simulink model "Ex6_6"  (Simulink 6.0)
settings: Solver=FixedStepDiscrete  SolverMode=SingleTasking  StartTime=0.0  StopTime=Ts*10  FixedStep=Ts  RelTol=1e-3  AbsTol=1e-6
values from neighbouring files (symbols this model uses):
  alpha1 = 1-1/Gain1    (= 0.99999)    [Ex6_6Launch.m]
  alpha2 = 1-1/Gain2    (= 0.99999)    [Ex6_6Launch.m]
  Ampl = 10^(Amp_dB/20)-pi/1024    (= 0.498119272052)    [Ex6_6Launch.m]
  finrad = Fin*2*pi    (= 882038.953034)    [Ex6_6Launch.m]
  GBW1 = 30000e6    (= 30000000000)    [Ex6_6Launch.m]
  GBW2 = 100e6    (= 100000000)    [Ex6_6Launch.m]
  sr1 = 79e6    (= 79000000)    [Ex6_6Launch.m]
  sr2 = 325e6    (= 325000000)    [Ex6_6Launch.m]
  Ts = 1/Fs    (= 2e-08)    [Ex6_6Launch.m]
undefined symbols (not defined in the file or in its folder): slew
settings Model: Creator=francomaloberti  LastModifiedBy=Cri  ExtModeAutoUpdateStatusClock=off
settings DataIOCC: LimitDataPoints=off  SignalLoggingName=sigsOut
settings OptimizationCC: BooleanDataType=off  InlineInvariantSignals=off
settings DebuggingCC: SolverPrmCheckMsg=none
settings HardwareCC: TargetUnknown=on

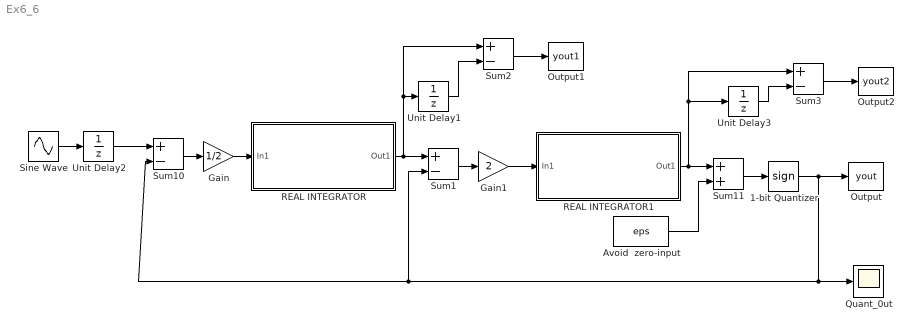
== system Ex6_6 ==
  1-bit Quantizer : Signum
  Avoid  zero-input : Constant  Value=eps
  Gain : Gain  Gain=1/2  SaturateOnIntegerOverflow=on
  Gain1 : Gain  Gain=2  SaturateOnIntegerOverflow=on
  Output : ToWorkspace  VariableName=yout  SampleTime=-1  SaveFormat=Array
  Output1 : ToWorkspace  VariableName=yout1  SampleTime=-1  SaveFormat=Array
  Output2 : ToWorkspace  VariableName=yout2  SampleTime=-1  SaveFormat=Array
  Quant_0ut : Scope
  REAL INTEGRATOR : Subsystem
      mask Display:
      | patch([10 40 10 10], [0 20 40 0],[1 0 1])
      | plot([10 40 10 10], [0 20 40 0])
      | plot([0 10], [20 20])
      | dpoly([0 1], [1 -1], 'z-')
      | port_label('input', 1, 'in')
  REAL INTEGRATOR1 : Subsystem
      mask Display:
      | patch([10 40 10 10], [0 20 40 0],[1 0 1])
      | plot([10 40 10 10], [0 20 40 0])
      | plot([0 10], [20 20])
      | dpoly([0 1], [1 -1], 'z-')
      | port_label('input', 1, 'in')
  Sine Wave : Sin  Amplitude=Ampl  Frequency=finrad  SampleTime=0
  Sum{1..3,10} (4 alike) : Sum  Inputs=+-  SaturateOnIntegerOverflow=on  InputSameDT=on
  Sum11 : Sum  SaturateOnIntegerOverflow=on  InputSameDT=on
  Unit Delay1 : UnitDelay  SampleTime=Ts
  Unit Delay2 : UnitDelay  SampleTime=Ts
  Unit Delay3 : UnitDelay  SampleTime=Ts
  wires:
  Sine Wave/1 -> Unit Delay2/1
  Unit Delay2/1 -> Sum10/1
  1-bit Quantizer/1 -> Quant_0ut/1, Sum10/2, Sum1/2, Output/1
  Sum10/1 -> Gain/1
  Gain/1 -> REAL INTEGRATOR/1(In1)
  Sum1/1 -> Gain1/1
  Gain1/1 -> REAL INTEGRATOR1/1(In1)
  REAL INTEGRATOR/1(Out1) -> Sum1/1, Unit Delay1/1, Sum2/1
  REAL INTEGRATOR1/1(Out1) -> Sum11/1, Unit Delay3/1, Sum3/1
  Sum11/1 -> 1-bit Quantizer/1
  Avoid  zero-input/1 -> Sum11/2
  Unit Delay1/1 -> Sum2/2
  Sum2/1 -> Output1/1
  Unit Delay3/1 -> Sum3/2
  Sum3/1 -> Output2/1

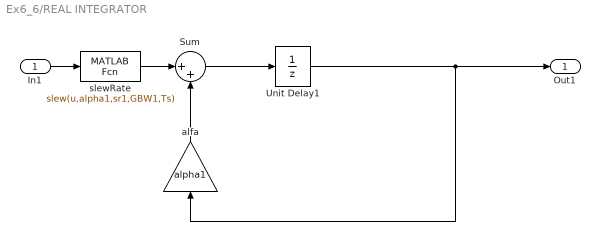
== system Ex6_6/REAL INTEGRATOR ==
  In1 : Inport  Port=1  LatchInput=off
  Sum : Sum  Inputs=|++  SaturateOnIntegerOverflow=on
  Unit Delay1 : UnitDelay  SampleTime=Ts
  alfa : Gain  Orientation=up  Gain=alpha1  SaturateOnIntegerOverflow=on
  slewRate : MATLABFcn  MATLABFcn=slew(u,alpha1,sr1,GBW1,Ts)
  Out1 : Outport
  wires:
  Sum/1 -> Unit Delay1/1
  In1/1 -> slewRate/1
  Unit Delay1/1 -> Out1/1, alfa/1
  slewRate/1 -> Sum/1
  alfa/1 -> Sum/2

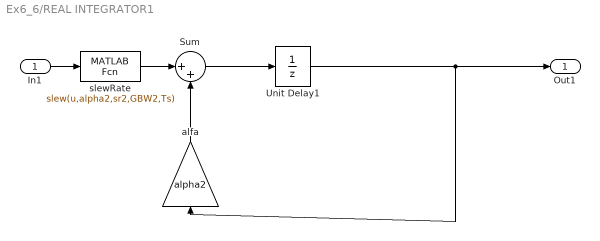
== system Ex6_6/REAL INTEGRATOR1 ==
  In1 : Inport  Port=1  LatchInput=off
  Sum : Sum  Inputs=|++  SaturateOnIntegerOverflow=on
  Unit Delay1 : UnitDelay  SampleTime=Ts
  alfa : Gain  Orientation=up  Gain=alpha2  SaturateOnIntegerOverflow=on
  slewRate : MATLABFcn  MATLABFcn=slew(u,alpha2,sr2,GBW2,Ts)
  Out1 : Outport
  wires:
  Sum/1 -> Unit Delay1/1
  In1/1 -> slewRate/1
  Unit Delay1/1 -> Out1/1, alfa/1
  slewRate/1 -> Sum/1
  alfa/1 -> Sum/2
